simulink model "x11untitled"  (R2023a)
settings: Solver=VariableStepAuto  StartTime=0.0  StopTime=10.0  RelTol=1e-3
settings Model: Creator=etoki  LastModifiedBy=etoki

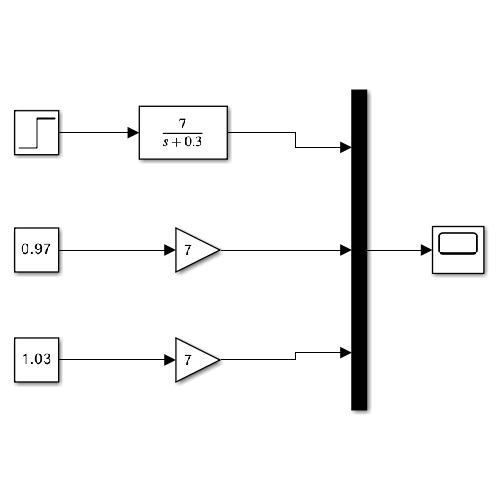
[thumbnail: Simulink's stored preview of the top-level diagram]
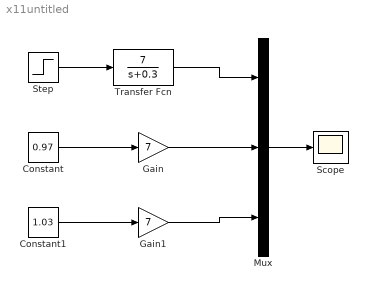
== system x11untitled ==
  Constant : Constant  Value=0.97
  Constant1 : Constant  Value=1.03
  Gain : Gain  Gain=7
  Gain1 : Gain  Gain=7
  Mux : Mux  Inputs=3
  Scope : Scope
  Step : Step  SampleTime=0
  Transfer Fcn : TransferFcn  Numerator=[7]  Denominator=[1 0.3]
  wires:
  Step/1 -> Transfer Fcn/1
  Constant/1 -> Gain/1
  Constant1/1 -> Gain1/1
  Mux/1 -> Scope/1
  Transfer Fcn/1 -> Mux/1
  Gain/1 -> Mux/2
  Gain1/1 -> Mux/3
